simulink model "MonopileSimulinkModelSFunc"  (R2022a)
settings: Solver=ode45  StartTime=0.0  StopTime=60  MaxStep=0.1  RelTol=1e-3
libraries: simulink x2
settings Model: Creator=jacobfontaine  LastModifiedBy=jacobfontaine

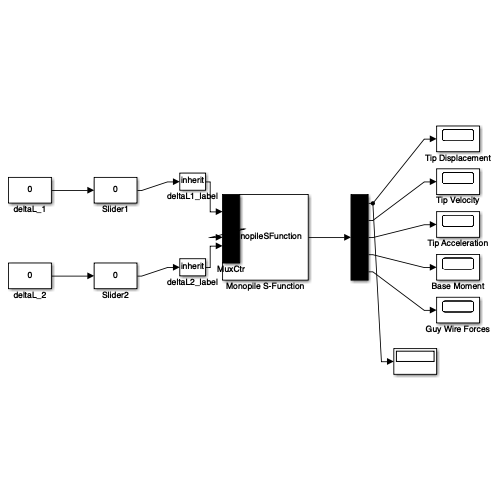
[thumbnail: Simulink's stored preview of the top-level diagram]
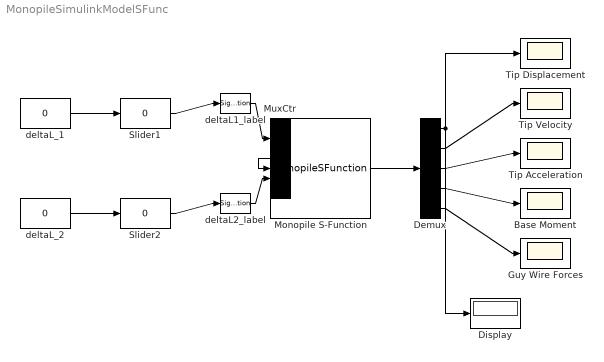
== system MonopileSimulinkModelSFunc ==
  Base Moment : Scope
  Demux : Demux  Outputs=5
  Display : Display
  Guy Wire Forces : Scope
  Monopile S-Function : S-Function  FunctionName=monopileSFunction  SFunctionDeploymentMode=off  EnableBusSupport=off
  MuxCtr : Mux  Inputs=2
  Slider1 : simulink/Math Operations/Slider Gain  gain=0  low=0  high=2
  Slider2 : simulink/Math Operations/Slider Gain  gain=0  low=0  high=2
  Tip Acceleration : Scope
  Tip Displacement : Scope
  Tip Velocity : Scope
  deltaL1_label : SignalSpecification
  deltaL2_label : SignalSpecification
  deltaL_1 : Constant  Value=0
  deltaL_2 : Constant  Value=0
  wires:
  deltaL_1/1 -> Slider1/1
  Slider1/1 -> deltaL1_label/1
  deltaL1_label/1 -> MuxCtr/1
  deltaL_2/1 -> Slider2/1
  Slider2/1 -> deltaL2_label/1
  deltaL2_label/1 -> MuxCtr/2
  MuxCtr/1 -> Monopile S-Function/1
  Monopile S-Function/1 -> Demux/1
  Demux/1 -> Tip Displacement/1, Display/1
  Demux/2 -> Tip Velocity/1
  Demux/3 -> Tip Acceleration/1
  Demux/4 -> Base Moment/1
  Demux/5 -> Guy Wire Forces/1
